simulink model "mainmodel"  (R2020a)
settings: Solver=VariableStepAuto  StartTime=0.0  StopTime=10.0  RelTol=1e-3
PreLoadFcn:
  | J = 0.00061;
  | Ke = 0.00637;
  | Kt = 0.2663;
  | Ra = 0.6187;
  | La = 2.62;
  | Kf = 0.00291;
  | Tou = 0.0781;
  | t = 10;
undefined symbols (not defined in the file): Kb
libraries: simulink x1
settings Model: Creator=Bhanu  LastModifiedBy=Bhanu

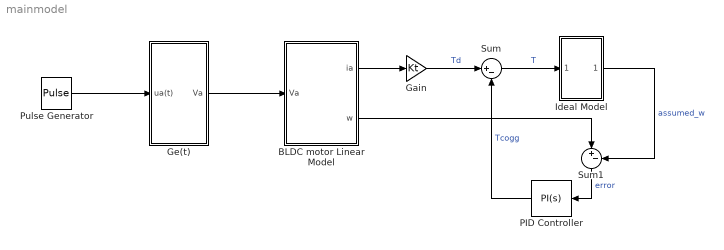
== system mainmodel ==
  BLDC motor Linear Model : Subsystem
  Gain : Gain  Gain=Kt
  Ge(t) : Subsystem
  Ideal Model : Subsystem
  PID Controller : simulink/Continuous/PID Controller  Controller=PI  Form=Parallel  TimeDomain=Continuous-time  UseExternalTs=off  SampleTime=-1  IntegratorMethod=Forward Euler  FilterMethod=Forward Euler  ControllerParametersSource=internal  P=1  I=1  D=0  UseFilter=on  N=100  TunerSelectOption=Transfer Function Based (PID Tuner App)  InitialConditionSource=internal  InitialConditionForIntegrator=0  InitialConditionForFilter=0  DifferentiatorICPrevScaledInput=0  ExternalReset=none  TrackingMode=off  Kt=1  LimitOutput=off  UpperSaturationLimit=inf  LowerSaturationLimit=-inf  LinearizeAsGain=on  AntiWindupMode=none  Kb=1  POutMin=[]  POutMax=[]  IOutMin=[]  IOutMax=[]  DOutMin=[]  DOutMax=[]  NOutMin=[]  NOutMax=[]  SumOutMin=[]  SumOutMax=[]  SaturationOutMin=[]  SaturationOutMax=[]  PParamMin=[]  PParamMax=[]  IParamMin=[]  IParamMax=[]  DParamMin=[]  DParamMax=[]  NParamMin=[]  NParamMax=[]  KbParamMin=[]  KbParamMax=[]  KtParamMin=[]  KtParamMax=[]  KbOutMin=[]  KbOutMax=[]  KtOutMin=[]  KtOutMax=[]  IntegratorOutMin=[]  IntegratorOutMax=[]  FilterOutMin=[]  FilterOutMax=[]  SumI1OutMin=[]  SumI1OutMax=[]  SumI2OutMin=[]  SumI2OutMax=[]  SumI3OutMin=[]  SumI3OutMax=[]  SumI4OutMin=[]  SumI4OutMax=[]  SumDOutMin=[]  SumDOutMax=[]  DifferentiatorOutMin=[]  DifferentiatorOutMax=[]  FilterDiffOutCoefMin=[]  FilterDiffOutCoefMax=[]  ReciprocalOutMin=[]  ReciprocalOutMax=[]  SumDenOutMin=[]  SumDenOutMax=[]  SumNumOutMin=[]  SumNumOutMax=[]  DivideOutMin=[]  DivideOutMax=[]  UdiffTsProdOutMin=[]  UdiffTsProdOutMax=[]  NTsProdOutMin=[]  NTsProdOutMax=[]  UintegralTsProdOutMin=[]  UintegralTsProdOutMax=[]  UngainTsProdOutMin=[]  UngainTsProdOutMax=[]  IntegratorContinuousStateAttributes=''  IntegratorStateMustResolveToSignalObject=off  IntegratorRTWStateStorageClass=Auto  FilterContinuousStateAttributes=''  FilterStateMustResolveToSignalObject=off  FilterRTWStateStorageClass=Auto  ParallelPVariant=InternalParameters  IdealPVariant=Disabled  IVariant=InternalParameters  DVariant=Disabled  IntegratorVariant=Continuous  SatVariant=Disabled  AWVariant=Passthrough  PCopyVariant=Disabled  TRVariant=Disabled  FdbkBlocksVariant=Forward  IdealPFdbkVariant=Disabled  SatFdbkVariant=Disabled  DerivativeFilterVariant=Disabled  NVariant=Disabled  NCopyVariant=Disabled_SignalSpec  FilterICVariant=Disabled  IntegratorICVariant=InternalICs  ExternalResetVariant=Disabled  TRSumVariant=Passthrough  SumFdbkVariant=Disabled  SumVariant=Sum_PI  TsampFilterVariant=InternalTs  TsampNgainVariant=Passthrough  TsampIntegralVariant=Passthrough
  Pulse Generator : DiscretePulseGenerator  PulseType=Time based  Period=10  PulseWidth=5
  Sum : Sum  Inputs=|+-
  Sum1 : Sum  Inputs=|+-
  wires:
  Ge(t)/1(Va) -> BLDC motor Linear Model/1(Va)
  Gain/1 -> Sum/1  "Td"
  Sum/1 -> Ideal Model/1(In1)  "T"
  Ideal Model/1(Out1) -> Sum1/2  "assumed_w"
  BLDC motor Linear Model/1(ia) -> Gain/1
  BLDC motor Linear Model/2(w) -> Sum1/1
  Sum1/1 -> PID Controller/1  "error"
  PID Controller/1 -> Sum/2  "Tcogg"
  Pulse Generator/1 -> Ge(t)/1(ua(t))

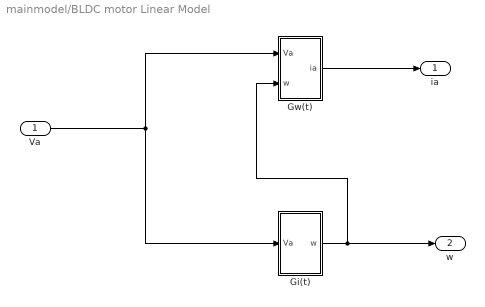
== system mainmodel/BLDC motor Linear Model ==
  Va : Inport
  Gi(t) : Subsystem
  Gw(t) : Subsystem
  ia : Outport
  w : Outport  Port=2
  wires:
  Va/1 -> Gw(t)/1(Va), Gi(t)/1(Va)
  Gi(t)/1(w) -> Gw(t)/2(w), w/1
  Gw(t)/1(ia) -> ia/1

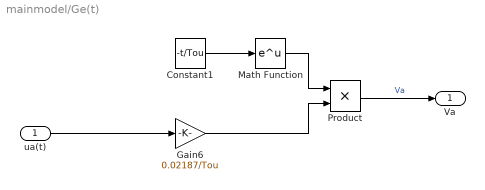
== system mainmodel/Ge(t) ==
  ua(t) : Inport
  Constant1 : Constant  Value=-t/Tou
  Gain6 : Gain  Gain=0.02187/Tou
  Math Function : Math  SaturateOnIntegerOverflow=on
  Product : Product
  Va : Outport
  wires:
  Constant1/1 -> Math Function/1
  Math Function/1 -> Product/1
  ua(t)/1 -> Gain6/1
  Gain6/1 -> Product/2
  Product/1 -> Va/1  "Va"

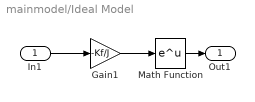
== system mainmodel/Ideal Model ==
  In1 : Inport
  Gain1 : Gain  Gain=-Kf/J
  Math Function : Math  SaturateOnIntegerOverflow=on
  Out1 : Outport
  wires:
  Gain1/1 -> Math Function/1
  Math Function/1 -> Out1/1
  In1/1 -> Gain1/1

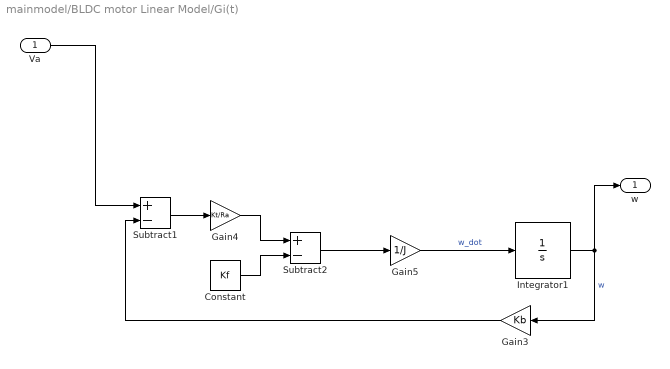
== system mainmodel/BLDC motor Linear Model/Gi(t) ==
  Va : Inport
  Constant : Constant  Value=Kf
  Gain3 : Gain  Gain=Kb
  Gain4 : Gain  Gain=Kt/Ra
  Gain5 : Gain  Gain=1/J
  Integrator1 : Integrator
  Subtract1 : Sum  Inputs=+-
  Subtract2 : Sum  Inputs=+-
  w : Outport
  wires:
  Integrator1/1 -> w/1, Gain3/1  "w"
  Subtract1/1 -> Gain4/1
  Constant/1 -> Subtract2/2
  Va/1 -> Subtract1/1
  Gain5/1 -> Integrator1/1  "w_dot"
  Subtract2/1 -> Gain5/1
  Gain4/1 -> Subtract2/1
  Gain3/1 -> Subtract1/2

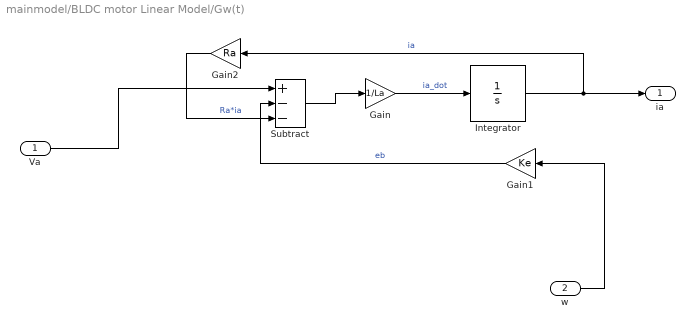
== system mainmodel/BLDC motor Linear Model/Gw(t) ==
  Va : Inport
  w : Inport  Port=2
  Gain : Gain  Gain=1/La
  Gain1 : Gain  Gain=Ke
  Gain2 : Gain  Gain=Ra
  Integrator : Integrator
  Subtract : Sum  Inputs=+--
  ia : Outport
  wires:
  w/1 -> Gain1/1
  Integrator/1 -> ia/1, Gain2/1  "ia"
  Gain1/1 -> Subtract/2  "eb"
  Va/1 -> Subtract/1
  Gain2/1 -> Subtract/3  "Ra*ia"
  Subtract/1 -> Gain/1
  Gain/1 -> Integrator/1  "ia_dot"
